simulink model "SWC_TRSP"  (R2020a)
settings: Solver=FixedStepDiscrete  StartTime=0.0  StopTime=0.15  FixedStep=0.0001  RelTol=1e-3
values from neighbouring files (symbols this model uses):
  CAL_TRSP_18VHSVoltCountTrh_s16 = 0.0    [SWC_TRSP_DataDictionary.sldd]
  CAL_TRSP_18VHSVoltDebTrh_s16 = 0.0    [SWC_TRSP_DataDictionary.sldd]
  CAL_TRSP_18VHSVoltErrRst_b = 0.0    [SWC_TRSP_DataDictionary.sldd]
  CAL_TRSP_18VHSVoltHiLim_u16 = 0.0    [SWC_TRSP_DataDictionary.sldd]
  CAL_TRSP_18VHSVoltLoLim_u16 = 0.0    [SWC_TRSP_DataDictionary.sldd]
  CAL_TRSP_1V8CPLDVoltCountTrh_s16 = 0.0    [SWC_TRSP_DataDictionary.sldd]
  CAL_TRSP_1V8CPLDVoltDebTrh_s16 = 0.0    [SWC_TRSP_DataDictionary.sldd]
  CAL_TRSP_1V8CPLDVoltErrRst_b = 0.0    [SWC_TRSP_DataDictionary.sldd]
  CAL_TRSP_1V8CPLDVoltHiLim_u16 = 0.0    [SWC_TRSP_DataDictionary.sldd]
  CAL_TRSP_1V8CPLDVoltLoLim_u16 = 0.0    [SWC_TRSP_DataDictionary.sldd]
  CAL_TRSP_3V3CPLDVoltCountTrh_s16 = 0.0    [SWC_TRSP_DataDictionary.sldd]
  CAL_TRSP_3V3CPLDVoltDebTrh_s16 = 0.0    [SWC_TRSP_DataDictionary.sldd]
  CAL_TRSP_3V3CPLDVoltErrRst_b = 0.0    [SWC_TRSP_DataDictionary.sldd]
  CAL_TRSP_3V3CPLDVoltHiLim_u16 = 0.0    [SWC_TRSP_DataDictionary.sldd]
  CAL_TRSP_3V3CPLDVoltLoLim_u16 = 0.0    [SWC_TRSP_DataDictionary.sldd]
  CAL_TRSP_AgTimecompCtl_u8 = 0.0    [SWC_TRSP_DataDictionary.sldd]
  CAL_TRSP_CurrRngCountTrh_s16 = 0.0    [SWC_TRSP_DataDictionary.sldd]
  CAL_TRSP_CurrRngDebTrh_s16 = 0.0    [SWC_TRSP_DataDictionary.sldd]
  CAL_TRSP_CurrRngErrRst_b = 0.0    [SWC_TRSP_DataDictionary.sldd]
  CAL_TRSP_CurrSumCountTrh_s16 = 0.0    [SWC_TRSP_DataDictionary.sldd]
  CAL_TRSP_CurrSumDebTrh_s16 = 0.0    [SWC_TRSP_DataDictionary.sldd]
  CAL_TRSP_CurrSumErrRst_b = 0.0    [SWC_TRSP_DataDictionary.sldd]
  CAL_TRSP_CurrSumLim_f32 = 0.0    [SWC_TRSP_DataDictionary.sldd]
  CAL_TRSP_Diff_UBR_SBCLim_f32 = 0.0    [SWC_TRSP_DataDictionary.sldd]
  CAL_TRSP_flgChangPha_b = 0.0    [SWC_TRSP_DataDictionary.sldd]
  CAL_TRSP_iPhasSensVoltCountTrh_s16 = 0.0    [SWC_TRSP_DataDictionary.sldd]
  CAL_TRSP_iPhasSensVoltDebTrh_s16 = 0.0    [SWC_TRSP_DataDictionary.sldd]
  CAL_TRSP_iPhasSensVoltErrRst_b = 0.0    [SWC_TRSP_DataDictionary.sldd]
  CAL_TRSP_iPhasSensVoltHiLim_u16 = 0.0    [SWC_TRSP_DataDictionary.sldd]
  CAL_TRSP_iPhasSensVoltLoLim_u16 = 0.0    [SWC_TRSP_DataDictionary.sldd]
  CAL_TRSP_iPhaUOffset_f32 = 0.0    [SWC_TRSP_DataDictionary.sldd]
  CAL_TRSP_iPhaVOffset_f32 = 0.0    [SWC_TRSP_DataDictionary.sldd]
  CAL_TRSP_iPhaWOffset_f32 = 0.0    [SWC_TRSP_DataDictionary.sldd]
  CAL_TRSP_iUCnvFac_f32 = 0.0    [SWC_TRSP_DataDictionary.sldd]
  CAL_TRSP_iVCnvFac_f32 = 0.0    [SWC_TRSP_DataDictionary.sldd]
  CAL_TRSP_iWCnvFac_f32 = 0.0    [SWC_TRSP_DataDictionary.sldd]
  CAL_TRSP_OfstErrRst_b = 0.0    [SWC_TRSP_DataDictionary.sldd]
  CAL_TRSP_OfstRngHiLim_f32 = 0.0    [SWC_TRSP_DataDictionary.sldd]
  CAL_TRSP_OfstRngLoLim_f32 = 0.0    [SWC_TRSP_DataDictionary.sldd]
  CAL_TRSP_ReqTrqCountTrh_s16 = 0.0    [SWC_TRSP_DataDictionary.sldd]
  CAL_TRSP_ReqTrqDebTrh_s16 = 0.0    [SWC_TRSP_DataDictionary.sldd]
  CAL_TRSP_ReqTrqErrRst_b = 0.0    [SWC_TRSP_DataDictionary.sldd]
  CAL_TRSP_ReqTrqHiLim_f32 = 0.0    [SWC_TRSP_DataDictionary.sldd]
  CAL_TRSP_ReqTrqLoLim_f32 = 0.0    [SWC_TRSP_DataDictionary.sldd]
  CAL_TRSP_RslvExciCountTrh_s16 = 0.0    [SWC_TRSP_DataDictionary.sldd]
  CAL_TRSP_RslvExciDebTrh_s16 = 0.0    [SWC_TRSP_DataDictionary.sldd]
  CAL_TRSP_RslvExciErrRst_b = 0.0    [SWC_TRSP_DataDictionary.sldd]
  CAL_TRSP_RslvMaxSele_u8 = 0.0    [SWC_TRSP_DataDictionary.sldd]
  CAL_TRSP_RslvMinSele_u8 = 0.0    [SWC_TRSP_DataDictionary.sldd]
  CAL_TRSP_RslvRngCosNHiLim_u16 = 0.0    [SWC_TRSP_DataDictionary.sldd]
  CAL_TRSP_RslvRngCosNLoLim_u16 = 0.0    [SWC_TRSP_DataDictionary.sldd]
  CAL_TRSP_RslvRngCosPHiLim_u16 = 0.0    [SWC_TRSP_DataDictionary.sldd]
  CAL_TRSP_RslvRngCosPLoLim_u16 = 0.0    [SWC_TRSP_DataDictionary.sldd]
  CAL_TRSP_RslvRngCountTrh_s16 = 0.0    [SWC_TRSP_DataDictionary.sldd]
  CAL_TRSP_RslvRngDebTrh_s16 = 0.0    [SWC_TRSP_DataDictionary.sldd]
  CAL_TRSP_RslvRngErrRst_b = 0.0    [SWC_TRSP_DataDictionary.sldd]
  CAL_TRSP_RslvRngExciHiLim_u16 = 0.0    [SWC_TRSP_DataDictionary.sldd]
  CAL_TRSP_RslvRngExciLoLim_u16 = 0.0    [SWC_TRSP_DataDictionary.sldd]
  CAL_TRSP_RslvRngSinNHiLim_u16 = 0.0    [SWC_TRSP_DataDictionary.sldd]
  CAL_TRSP_RslvRngSinNLoLim_u16 = 0.0    [SWC_TRSP_DataDictionary.sldd]
  CAL_TRSP_RslvRngSinPHiLim_u16 = 0.0    [SWC_TRSP_DataDictionary.sldd]
  CAL_TRSP_RslvRngSinPLoLim_u16 = 0.0    [SWC_TRSP_DataDictionary.sldd]
  CAL_TRSP_RslvSensVoltCountTrh_s16 = 0.0    [SWC_TRSP_DataDictionary.sldd]
  CAL_TRSP_RslvSensVoltDebTrh_s16 = 0.0    [SWC_TRSP_DataDictionary.sldd]
  CAL_TRSP_RslvSensVoltErrRst_b = 0.0    [SWC_TRSP_DataDictionary.sldd]
  CAL_TRSP_RslvSensVoltHiLim_u16 = 0.0    [SWC_TRSP_DataDictionary.sldd]
  CAL_TRSP_RslvSensVoltLoLim_u16 = 0.0    [SWC_TRSP_DataDictionary.sldd]
  CAL_TRSP_RslvSqrtCountTrh_s16 = 0.0    [SWC_TRSP_DataDictionary.sldd]
  CAL_TRSP_RslvSqrtDebTrh_s16 = 0.0    [SWC_TRSP_DataDictionary.sldd]
  CAL_TRSP_RslvSqrtErrRst_b = 0.0    [SWC_TRSP_DataDictionary.sldd]
  CAL_TRSP_RslvSqrtHiLim_u16 = 0.0    [SWC_TRSP_DataDictionary.sldd]
  CAL_TRSP_RslvSqrtLoLim_u16 = 0.0    [SWC_TRSP_DataDictionary.sldd]
  CAL_TRSP_SpeedCtlMode_u8 = 0.0    [SWC_TRSP_DataDictionary.sldd]
  CAL_TRSP_TorqueCtlMode_u8 = 0.0    [SWC_TRSP_DataDictionary.sldd]
  CAL_TRSP_UB_SBCCnvFac_f32 = 0.0    [SWC_TRSP_DataDictionary.sldd]
  CAL_TRSP_UBRVoltCountTrh_s16 = 0.0    [SWC_TRSP_DataDictionary.sldd]
  CAL_TRSP_UBRVoltDebTrh_s16 = 0.0    [SWC_TRSP_DataDictionary.sldd]
  CAL_TRSP_UBRVoltErrRst_b = 0.0    [SWC_TRSP_DataDictionary.sldd]
  CAL_TRSP_UBRWIDECnvFac_f32 = 0.0    [SWC_TRSP_DataDictionary.sldd]
  CAL_TRSP_UCurrRngHiLim_f32 = 0.0    [SWC_TRSP_DataDictionary.sldd]
  CAL_TRSP_UCurrRngLoLim_f32 = 0.0    [SWC_TRSP_DataDictionary.sldd]
  CAL_TRSP_VCurrRngHiLim_f32 = 0.0    [SWC_TRSP_DataDictionary.sldd]
  CAL_TRSP_VCurrRngLoLim_f32 = 0.0    [SWC_TRSP_DataDictionary.sldd]
  CAL_TRSP_WCurrRngHiLim_f32 = 0.0    [SWC_TRSP_DataDictionary.sldd]
  CAL_TRSP_WCurrRngLoLim_f32 = 0.0    [SWC_TRSP_DataDictionary.sldd]
  GLB_TRSP_CircAge_f32 = 0.0    [SWC_TRSP_DataDictionary.sldd]
  GLB_TRSP_MotorPole_u8 = 0.0    [SWC_TRSP_DataDictionary.sldd]
  GLB_TRSP_Sixty_f32 = 0.0    [SWC_TRSP_DataDictionary.sldd]
libraries: simulink x22
(part 11 of 13)

== system SWC_TRSP/SWC_TRSP_100us_sys/UBRVoltChk/UBRVoltCompChk ==
  TRSP_UBRWIDE : Inport
  TRSP_UB_SBC : Inport  Port=2
  Abs : Abs
  Add : Sum  Inputs=+-
  CAL_TOM_CurrSumLim_f32 : Constant  Value=CAL_TRSP_Diff_UBR_SBCLim_f32
  Relational Operator : RelationalOperator  OutDataTypeStr=boolean  RndMeth=Simplest
  TRSP_UBRVoltChkRslt : Outport
  wires:
  Add/1 -> Abs/1  "VAR_TRSP_Diff_UBR_SBC_f32"
  Abs/1 -> Relational Operator/1
  CAL_TOM_CurrSumLim_f32/1 -> Relational Operator/2
  Relational Operator/1 -> TRSP_UBRVoltChkRslt/1
  TRSP_UB_SBC/1 -> Add/2
  TRSP_UBRWIDE/1 -> Add/1

== system SWC_TRSP/SWC_TRSP_100us_sys/UBRVoltChk/UBR_SBCVoltCalc ==
  L2Sampling_UBRWIDE_MON : Inport
  L2Sampling_UB_SBC_MON : Inport  Port=2
  CAL_CSP_iUCnvFac_f32 : Constant  Value=CAL_TRSP_UBRWIDECnvFac_f32
  CAL_MCF_iWCnvFac_f32 : Constant  Value=CAL_TRSP_UB_SBCCnvFac_f32
  Product : Product
  Product2 : Product
  TRSP_UBRWIDE : Outport  VectorParamsAs1DForOutWhenUnconnected=off
  TRSP_UB_SBC : Outport  Port=2  VectorParamsAs1DForOutWhenUnconnected=off
  wires:
  Product/1 -> TRSP_UBRWIDE/1
  L2Sampling_UB_SBC_MON/1 -> Product2/1
  CAL_MCF_iWCnvFac_f32/1 -> Product2/2
  L2Sampling_UBRWIDE_MON/1 -> Product/1
  CAL_CSP_iUCnvFac_f32/1 -> Product/2
  Product2/1 -> TRSP_UB_SBC/1

== system SWC_TRSP/SWC_TRSP_100us_sys/iPhasSensVoltChk/Debouncer12 ==
  note: 1
  note: 1
  note: 0
  BooleanIN : Inport
  Rst : Inport  Port=2
  CountTrh : Inport  Port=3
  DebTrh : Inport  Port=4
  Add : Sum
  Boolean_ZERO : Constant  Value=0  OutDataTypeStr=boolean
  Compare To Zero : simulink/Logic and Bit Operations/Compare To Zero  relop===  OutDataTypeStr=boolean
  Constant : Constant  Value=0  OutDataTypeStr=int16
  Constant1 : Constant  Value=0  OutDataTypeStr=int16
  Count : Subsystem
  Delay1 : Delay  DelayLength=1
  Delay2 : Delay  DelayLength=1
  Logical Operator : Logic  Operator=OR  AllPortsSameDT=off  OutDataTypeStr=boolean
  Logical Operator1 : Logic  Operator=OR  AllPortsSameDT=off  OutDataTypeStr=boolean
  Relational Operator : RelationalOperator  OutDataTypeStr=boolean  RndMeth=Simplest
  Switch : Switch  Criteria=u2 > Threshold
  Switch1 : Switch  Criteria=u2 ~= 0
  Switch2 : Switch  Criteria=u2 > Threshold
  Unit Delay1 : UnitDelay  SampleTime=-1  HasFrameUpgradeWarning=on
  OutLock : Outport  VectorParamsAs1DForOutWhenUnconnected=off
  wires:
  Delay2/1 -> Switch2/3
  CountTrh/1 -> Count/1(CountTrh)
  Logical Operator1/1 -> Delay1/1
  Delay1/1 -> Count/Enable, Logical Operator1/1
  Switch2/1 -> Add/2
  Constant/1 -> Switch2/1
  Compare To Zero/1 -> Switch2/2
  Count/1(Count) -> Compare To Zero/1
  Logical Operator/1 -> OutLock/1, Unit Delay1/1
  Boolean_ZERO/1 -> Switch1/1
  Rst/1 -> Switch1/2
  Switch1/1 -> Logical Operator/2
  Unit Delay1/1 -> Switch1/3
  BooleanIN/1 -> Logical Operator1/2, Add/1
  Relational Operator/1 -> Switch/2, Logical Operator/1
  DebTrh/1 -> Relational Operator/2
  Switch/1 -> Delay2/1
  Add/1 -> Switch/3, Relational Operator/1
  Constant1/1 -> Switch/1

== system SWC_TRSP/SWC_TRSP_100us_sys/iPhasSensVoltChk/RngChk ==
  TRSP_RngChkVal : Inport
  TRSP_HiTrh : Inport  Port=2
  TRSP_LoTrh : Inport  Port=3
  Logical Operator : Logic  Operator=OR  AllPortsSameDT=off  OutDataTypeStr=boolean
  Relational Operator : RelationalOperator  Operator=<=  OutDataTypeStr=boolean  RndMeth=Simplest
  Relational Operator1 : RelationalOperator  OutDataTypeStr=boolean  RndMeth=Simplest
  TRSP_RngChkRslt : Outport
  wires:
  Relational Operator1/1 -> Logical Operator/1
  TRSP_LoTrh/1 -> Relational Operator/2
  TRSP_RngChkVal/1 -> Relational Operator1/1, Relational Operator/1
  Logical Operator/1 -> TRSP_RngChkRslt/1
  TRSP_HiTrh/1 -> Relational Operator1/2
  Relational Operator/1 -> Logical Operator/2

== system SWC_TRSP/SWC_TRSP_10ms_sys/CANSigChk/Debouncer15 ==
  note: 0
  note: 1
  note: 1
  BooleanIN : Inport
  Rst : Inport  Port=2
  CountTrh : Inport  Port=3
  DebTrh : Inport  Port=4
  Add : Sum
  Boolean_ZERO : Constant  Value=0  OutDataTypeStr=boolean
  Compare To Zero : simulink/Logic and Bit Operations/Compare To Zero  relop===  OutDataTypeStr=boolean
  Constant : Constant  Value=0  OutDataTypeStr=int16
  Constant1 : Constant  Value=0  OutDataTypeStr=int16
  Count : Subsystem
  Delay1 : Delay  DelayLength=1
  Delay2 : Delay  DelayLength=1
  Logical Operator : Logic  Operator=OR  AllPortsSameDT=off  OutDataTypeStr=boolean
  Logical Operator1 : Logic  Operator=OR  AllPortsSameDT=off  OutDataTypeStr=boolean
  Relational Operator : RelationalOperator  OutDataTypeStr=boolean  RndMeth=Simplest
  Switch : Switch  Criteria=u2 > Threshold
  Switch1 : Switch  Criteria=u2 ~= 0
  Switch2 : Switch  Criteria=u2 > Threshold
  Unit Delay1 : UnitDelay  SampleTime=-1  HasFrameUpgradeWarning=on
  OutLock : Outport  VectorParamsAs1DForOutWhenUnconnected=off
  wires:
  Constant1/1 -> Switch/1
  Add/1 -> Relational Operator/1, Switch/3
  Switch/1 -> Delay2/1
  DebTrh/1 -> Relational Operator/2
  Relational Operator/1 -> Logical Operator/1, Switch/2
  BooleanIN/1 -> Add/1, Logical Operator1/2
  Unit Delay1/1 -> Switch1/3
  Switch1/1 -> Logical Operator/2
  Rst/1 -> Switch1/2
  Boolean_ZERO/1 -> Switch1/1
  Logical Operator/1 -> Unit Delay1/1, OutLock/1
  Count/1(Count) -> Compare To Zero/1
  Compare To Zero/1 -> Switch2/2
  Constant/1 -> Switch2/1
  Switch2/1 -> Add/2
  Delay1/1 -> Logical Operator1/1, Count/Enable
  Logical Operator1/1 -> Delay1/1
  CountTrh/1 -> Count/1(CountTrh)
  Delay2/1 -> Switch2/3

== system SWC_TRSP/SWC_TRSP_10ms_sys/CANSigChk/RngChk2 ==
  TRSP_RngChkVal : Inport
  TRSP_HiTrh : Inport  Port=2
  TRSP_LoTrh : Inport  Port=3
  Logical Operator : Logic  Operator=OR  AllPortsSameDT=off  OutDataTypeStr=boolean
  Relational Operator : RelationalOperator  Operator=<=  OutDataTypeStr=boolean  RndMeth=Simplest
  Relational Operator1 : RelationalOperator  OutDataTypeStr=boolean  RndMeth=Simplest
  TRSP_RngChkRslt : Outport
  wires:
  Relational Operator1/1 -> Logical Operator/1
  TRSP_LoTrh/1 -> Relational Operator/2
  TRSP_RngChkVal/1 -> Relational Operator1/1, Relational Operator/1
  Logical Operator/1 -> TRSP_RngChkRslt/1
  TRSP_HiTrh/1 -> Relational Operator1/2
  Relational Operator/1 -> Logical Operator/2

== system SWC_TRSP/SWC_TRSP_10ms_sys/Debouncer/Subsystem ==
  CountTrh : Inport
  Enable : EnablePort
  Add : Sum
  Constant : Constant  OutDataTypeStr=int16
  Constant1 : Constant  Value=0  OutDataTypeStr=int16
  Delay : Delay  DelayLength=1
  Relational Operator : RelationalOperator  OutDataTypeStr=boolean  RndMeth=Simplest
  Switch : Switch  Criteria=u2 > Threshold
  Count : Outport
  wires:
  Delay/1 -> Add/2
  CountTrh/1 -> Relational Operator/2
  Constant1/1 -> Switch/1
  Add/1 -> Switch/3, Relational Operator/1
  Relational Operator/1 -> Switch/2
  Constant/1 -> Add/1
  Switch/1 -> Count/1, Delay/1

== system SWC_TRSP/SWC_TRSP_1ms_sys/Debouncer/Subsystem ==
  CountTrh : Inport
  Enable : EnablePort
  Add : Sum
  Constant : Constant  OutDataTypeStr=int16
  Constant1 : Constant  Value=0  OutDataTypeStr=int16
  Delay : Delay  DelayLength=1
  Relational Operator : RelationalOperator  OutDataTypeStr=boolean  RndMeth=Simplest
  Switch : Switch  Criteria=u2 > Threshold
  Count : Outport
  wires:
  Switch/1 -> Delay/1, Count/1
  Constant/1 -> Add/1
  Relational Operator/1 -> Switch/2
  Add/1 -> Relational Operator/1, Switch/3
  Constant1/1 -> Switch/1
  CountTrh/1 -> Relational Operator/2
  Delay/1 -> Add/2

== system SWC_TRSP/SWC_TRSP_1ms_sys/OfstAgChk/OfstChk ==
  NvM_AngAutoClbOffset : Inport
  Enable : EnablePort
  CAL_TOM_OfstErrRst_b : Constant  Value=CAL_TRSP_OfstErrRst_b  OutDataTypeStr=boolean
  CAL_TOM_OfstRngHiLim_f32 : Constant  Value=CAL_TRSP_OfstRngHiLim_f32  OutDataTypeStr=single
  CAL_TOM_OfstRngLoLim_f32 : Constant  Value=CAL_TRSP_OfstRngLoLim_f32  OutDataTypeStr=single
  Lock : Subsystem  TreatAsAtomicUnit=on
      settings: RTWSystemCode=Nonreusable function
  OfstRngChk : Subsystem  TreatAsAtomicUnit=on
  TRSP_OfstRngErr : Outport
  wires:
  OfstRngChk/1(TRSP_OfstRngChkRslt) -> Lock/1(BooleanIN)  "VAR_TRSP_OfstRngChkRslt_b"
  NvM_AngAutoClbOffset/1 -> OfstRngChk/1(TRSP_OfstRngChkVal)
  Lock/1(OutLock) -> TRSP_OfstRngErr/1  "VAR_TRSP_OfstRngErr_b"
  CAL_TOM_OfstErrRst_b/1 -> Lock/2(Rst)
  CAL_TOM_OfstRngHiLim_f32/1 -> OfstRngChk/2(TRSP_HiTrh)
  CAL_TOM_OfstRngLoLim_f32/1 -> OfstRngChk/3(TRSP_LoTrh)

== system SWC_TRSP/SWC_TRSP_1ms_sys/OfstAgChk/OfstChkEnable ==
  L2Com_ModeReq : Inport
  Add : Sum
  CAL_TOM_SpeedCtlMode_u2 : Constant  Value=CAL_TRSP_TorqueCtlMode_u8  OutDataTypeStr=uint8
  CAL_TOM_SpeedCtlMode_u3 : Constant  Value=CAL_TRSP_SpeedCtlMode_u8  OutDataTypeStr=uint8
  Compare To Constant : simulink/Logic and Bit Operations/Compare To Constant  relop===  const=1  OutDataTypeStr=boolean
  Constant : Constant  OutDataTypeStr=uint8
  Delay : Delay  DelayLength=1
  Logical Operator : Logic  Operator=OR  AllPortsSameDT=off  OutDataTypeStr=boolean
  Logical Operator2 : Logic  AllPortsSameDT=off  OutDataTypeStr=boolean
  Relational Operator3 : RelationalOperator  Operator===  OutDataTypeStr=boolean  RndMeth=Simplest
  Relational Operator4 : RelationalOperator  Operator===  OutDataTypeStr=boolean  RndMeth=Simplest
  Enable : Outport
  wires:
  Relational Operator4/1 -> Logical Operator/1
  Logical Operator/1 -> Logical Operator2/2
  L2Com_ModeReq/1 -> Relational Operator3/1, Relational Operator4/1
  Logical Operator2/1 -> Enable/1
  Relational Operator3/1 -> Logical Operator/2
  CAL_TOM_SpeedCtlMode_u3/1 -> Relational Operator4/2
  Compare To Constant/1 -> Logical Operator2/1
  CAL_TOM_SpeedCtlMode_u2/1 -> Relational Operator3/2
  Constant/1 -> Add/2
  Add/1 -> Compare To Constant/1, Delay/1
  Delay/1 -> Add/1

== system SWC_TRSP/SWC_TRSP_100us_sys/18VHSVoltChk/Debouncer11/Count ==
  CountTrh : Inport
  Enable : EnablePort
  Add : Sum
  Constant : Constant  OutDataTypeStr=int16
  Constant1 : Constant  Value=0  OutDataTypeStr=int16
  Delay : Delay  DelayLength=1
  Relational Operator : RelationalOperator  OutDataTypeStr=boolean  RndMeth=Simplest
  Switch : Switch  Criteria=u2 > Threshold
  Count : Outport
  wires:
  Delay/1 -> Add/2
  CountTrh/1 -> Relational Operator/2
  Constant1/1 -> Switch/1
  Add/1 -> Switch/3, Relational Operator/1
  Relational Operator/1 -> Switch/2
  Constant/1 -> Add/1
  Switch/1 -> Count/1, Delay/1
